simulink library "Feeder2_lib"  (Simulink 8.1)
settings: Solver=ode45  StartTime=0.0  StopTime=10.0  RelTol=1e-3
values from neighbouring files (symbols this model uses):
  DER_REL = xlsread('DER_relay.xlsx')    [relay_settings_init.m]
  Ts = 100E-6    (= 0.0001)    [BANSHEE_init.m]    (also in Ghost_init.m)
undefined symbols (not defined in the file or in its folder): CBID, Left, type, V
libraries: breaker_lib x22, powerlib x13, cables_lib x12, transformer_lib x10, Load_lib x8, ssn_lib x7, BESS_lib x2, relay_modbus_lib x2, rtio_generic_modbus x2, rtlab x2
settings Model: Creator=re25624  LastModifiedBy=MGC3

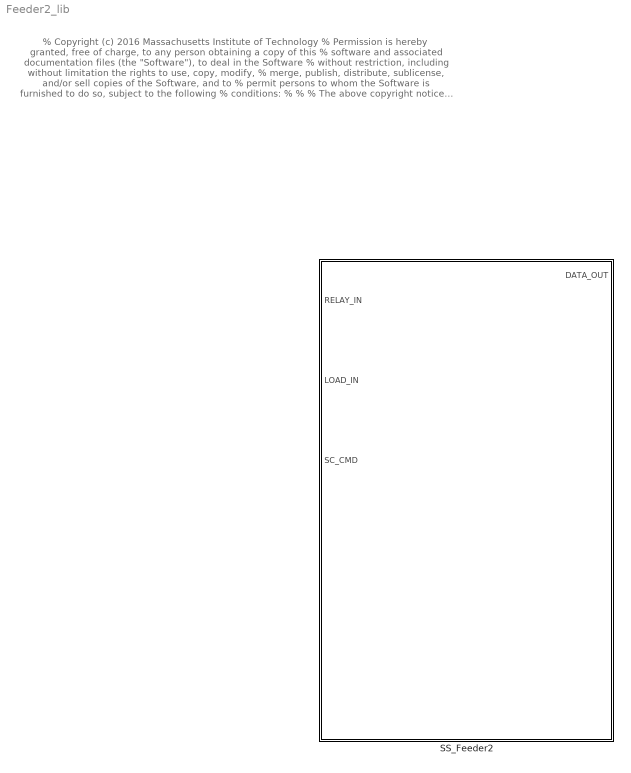
== system Feeder2_lib ==
  note: % Copyright (c) 2016 Massachusetts Institute of Technology
      | % Permission is hereby granted, free of charge, to any person obtaining a copy of this
      | % software and associated documentation files (the "Software"), to deal in the Software
      | % without restriction, including without limitation the rights to use, copy, modify,
      | % merge, publish, distribute, sublicense, and/or sell copies of the Software, and to
      | % permit persons to whom the Software is furnished to do so, subject to the following
      | % conditions:
      | %
      | %
      | % The above copyright notice and this permission notice shall be included in
      | % all copies or substantial portions of the Software.
      | %
      | % THE SOFTWARE IS PROVIDED "AS IS", WITHOUT WARRANTY OF ANY KIND, EXPRESS OR IMPLIED,
      | % INCLUDING BUT NOT LIMITED TO THE WARRANTIES OF MERCHANTABILITY, FITNESS FOR A
      | % PARTICULAR PURPOSE AND NONINFRINGEMENT. IN NO EVENT SHALL THE AUTHORS OR COPYRIGHT
      | % HOLDERS BE LIABLE FOR ANY CLAIM, DAMAGES OR OTHER LIABILITY, WHETHER IN AN ACTION
      | % OF CONTRACT, TORT OR OTHERWISE, ARISING FROM, OUT OF OR IN CONNECTION WITH THE
      | % SOFTWARE OR THE USE OR OTHER DEALINGS IN THE SOFTWARE.
      | %
      | %
      | %%
  SS_Feeder2 : Subsystem

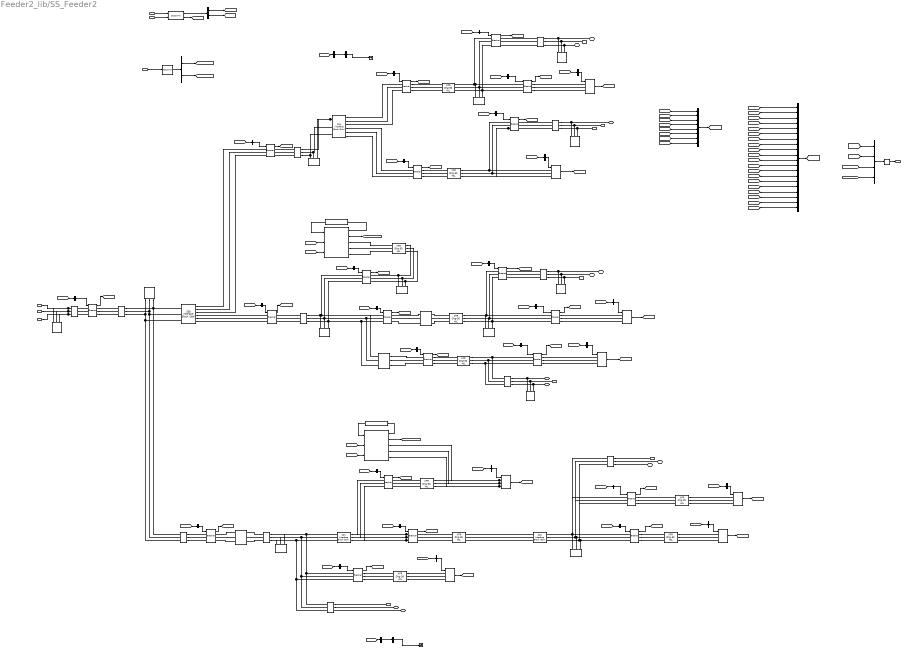
== system Feeder2_lib/SS_Feeder2 ==
  note: Fault6:
      | Fault Resistance: 0.1Ohm
      | Ground Resistance: 1.73Ohm
      | Snubber resistance: 1E6:
  note: Fault5:
      | Fault Resistance: 0.1Ohm
      | Ground Resistance: 1.73Ohm
      | Snubber resistance: 1E6:
  note: BESS SYSTEM
  note: % Copyright (c) 2016 Massachusetts Institute of Technology
      | % Permission is hereby granted, free of charge, to any person obtaining a copy of this
      | % software and associated documentation files (the "Software"), to deal in the Software
      | % without restriction, including without limitation the rights to use, copy, modify,
      | % merge, publish, distribute, sublicense, and/or sell copies of the Software, and to
      | % permit persons to whom the Software is furnished to do so, subject to the following
      | % conditions:
      | %
      | %
      | % The above copyright notice and this permission notice shall be included in
      | % all copies or substantial portions of the Software.
      | %
      | % THE SOFTWARE IS PROVIDED "AS IS", WITHOUT WARRANTY OF ANY KIND, EXPRESS OR IMPLIED,
      | % INCLUDING BUT NOT LIMITED TO THE WARRANTIES OF MERCHANTABILITY, FITNESS FOR A
      | % PARTICULAR PURPOSE AND NONINFRINGEMENT. IN NO EVENT SHALL THE AUTHORS OR COPYRIGHT
      | % HOLDERS BE LIABLE FOR ANY CLAIM, DAMAGES OR OTHER LIABILITY, WHETHER IN AN ACTION
      | % OF CONTRACT, TORT OR OTHERWISE, ARISING FROM, OUT OF OR IN CONNECTION WITH THE
      | % SOFTWARE OR THE USE OR OTHER DEALINGS IN THE SOFTWARE.
      | %
      | %
      | %%
  note: connect to F1
  note: PV SYSTEM
  note: connect to F3
  note: connect to F3
  note: connect to F3
  note: connect to F1
  note: connect to F1
  RELAY_IN : Inport
  LOAD_IN : Inport  Port=2
  SC_CMD : Inport  Port=3
  1000 kVA1 : transformer_lib/XFR DYg-30 HIL  Rating=1000  Vp=13800  Vs=480  Z=5.56  XR=4.49
  1000 kVA2 : transformer_lib/XFR DYg-30 HIL  Rating=1000  Vp=4160  Vs=480  Z=5.56  XR=5.49
  1500 kVA : transformer_lib/XFR DYg-30 HIL  Rating=1500  Vp=4160  Vs=480  Z=5.56  XR=5.51
  2000 kVA2 : transformer_lib/XFR DYg-30 HIL  Rating=2000  Vp=13800  Vs=480  Z=5.75  XR=5.7
  2000 kVA3 : transformer_lib/XFR DYg-30 HIL  Rating=2000  Vp=13800  Vs=480  Z=5.75  XR=5.7
  2500 kVA : transformer_lib/XFR DYg-30 HIL  Rating=2500  Vp=13800  Vs=480  Z=5.56  XR=5.52
  2500 kVA1 : transformer_lib/XFR DYg-30 HIL  Rating=2500  Vp=13800  Vs=480  Z=5.56  XR=5.52
  3750 kVA : transformer_lib/XFR DYg-30 HIL  Rating=3750  Vp=13800  Vs=4160  Z=4.75  XR=11.4
  4/0AWG-Mutual : cables_lib/4//0AWG-Mutual  length=10  par_sets=1  ratio=3
  448 kvar inductor at 13.8kV  to cancel kvar produced by the stublines1 : powerlib/Elements/Three-Phase Parallel RLC Load  LConnTagsString=A|B|C  Configuration=Y (grounded)  NominalVoltage=13800  NominalFrequency=60  ActivePower=10e3  InductivePower=448e3  CapacitivePower=0  Measurements=None  LoadType=constant Z
  500 kVA : transformer_lib/XFR DYg-30 HIL  Rating=500  Vp=13800  Vs=208  Z=5  XR=4.9
  5000 kVA : transformer_lib/XFR DYg-30 HIL  Rating=5000  Vp=13800  Vs=480  Z=3  XR=5.44
  500kcmil-Mutual4 : cables_lib/500kcmil-Mutual  length=10  par_sets=1  ratio=3
  500kcmil-Mutual5 : cables_lib/500kcmil-Mutual  length=1000  par_sets=1  ratio=3
  500kcmil-Mutual8 : cables_lib/500kcmil-Mutual  length=100  par_sets=1  ratio=3
  6 kvar inductor at 480V  to cancel kvar produced by the stublines1 : powerlib/Elements/Three-Phase Parallel RLC Load  LConnTagsString=A|B|C  Configuration=Y (grounded)  NominalVoltage=480  NominalFrequency=60  ActivePower=1e3  InductivePower=6e3  CapacitivePower=0  Measurements=None  LoadType=constant Z
  6 kvar inductor at 480V  to cancel kvar produced by the stublines2 : powerlib/Elements/Three-Phase Parallel RLC Load  LConnTagsString=A|B|C  Configuration=Y (grounded)  NominalVoltage=480  NominalFrequency=60  ActivePower=1e3  InductivePower=6e3  CapacitivePower=0  Measurements=None  LoadType=constant Z
  6 kvar inductor at 480V  to cancel kvar produced by the stublines3 : powerlib/Elements/Three-Phase Parallel RLC Load  LConnTagsString=A|B|C  Configuration=Y (grounded)  NominalVoltage=480  NominalFrequency=60  ActivePower=1  InductivePower=6e3  CapacitivePower=0  Measurements=None  LoadType=constant Z
  6 kvar inductor at 480V  to cancel kvar produced by the stublines4 : powerlib/Elements/Three-Phase Parallel RLC Load  LConnTagsString=A|B|C  Configuration=Y (grounded)  NominalVoltage=480  NominalFrequency=60  ActivePower=1  InductivePower=9e3  CapacitivePower=0  Measurements=None  LoadType=constant Z
  Bus Creator2 : BusCreator
  Bus Creator3 : BusCreator  Inputs=8
  Bus Creator5 : BusCreator  Inputs=20
  Bus Selector1 : BusSelector  OutputSignals=F2_CB_4
  Bus Selector10 : BusSelector  OutputSignals=I4
  Bus Selector11 : BusSelector  OutputSignals=F2_CB_11
  Bus Selector12 : BusSelector  OutputSignals=F2_CB_15
  Bus Selector13 : BusSelector  OutputSignals=F2_CB_3
  Bus Selector14 : BusSelector  OutputSignals=F2_CB_14
  Bus Selector15 : BusSelector  OutputSignals=F2_CB_17
  Bus Selector16 : BusSelector  OutputSignals=F2_CB_16
  Bus Selector17 : BusSelector  OutputSignals=F2_CB_13
  Bus Selector18 : BusSelector  OutputSignals=F2_CB_10
  Bus Selector19 : BusSelector  OutputSignals=F2_CB_9
  Bus Selector2 : BusSelector  OutputSignals=F2_CB_2
  Bus Selector20 : BusSelector  OutputSignals=F2_CB_12
  Bus Selector21 : BusSelector  OutputSignals=F2_CB_5
  Bus Selector22 : BusSelector  OutputSignals=F2_CB_7
  Bus Selector23 : BusSelector  OutputSignals=F2_CB_8
  Bus Selector24 : BusSelector  OutputSignals=F2_CB_6
  Bus Selector25 : BusSelector  OutputSignals=F2_CB_1
  Bus Selector26 : BusSelector  OutputSignals=F2_CB_18
  Bus Selector27 : BusSelector  OutputSignals=F2_CB_19
  Bus Selector28 : BusSelector  OutputSignals=ESS1_ctrl,PV1_ctrl
  Bus Selector29 : BusSelector  OutputSignals=fault
  Bus Selector3 : BusSelector  OutputSignals=P5
  Bus Selector30 : BusSelector  OutputSignals=LoadProfile,TestSeq
  Bus Selector31 : BusSelector  OutputSignals=loc6
  Bus Selector32 : BusSelector  OutputSignals=fault
  Bus Selector33 : BusSelector  OutputSignals=loc5
  Bus Selector36 : BusSelector  OutputSignals=F2_PCC
  Bus Selector4 : BusSelector  OutputSignals=C4
  Bus Selector5 : BusSelector  OutputSignals=I5
  Bus Selector6 : BusSelector  OutputSignals=P2
  Bus Selector7 : BusSelector  OutputSignals=C3
  Bus Selector8 : BusSelector  OutputSignals=P3
  Bus Selector9 : BusSelector  OutputSignals=I3
  C{1..2,204..206} (5 alike) : cables_lib/500kcmil-Mutual  length=10  par_sets=1  ratio=3
  C201 : cables_lib/4//0AWG-Mutual  length=5500  par_sets=1  ratio=3
  C202 : cables_lib/500kcmil-Mutual  length=2000  par_sets=1  ratio=3
  C203 : cables_lib/500kcmil-Mutual  length=3000  par_sets=1  ratio=3
  Critical_3 : Load_lib/Dynamic_Load  V=480  kVA=1000  PF=0.9  Ts=Ts
  Critical_4 : Load_lib/Dynamic_Load  V=480  kVA=1000  PF=0.9  Ts=Ts
  ESS1 : Subsystem
  ESS1_Modbus : rtio_generic_modbus/Modbus device  conf_name=ESS1_modbus.opal  conf_name_mask=ESS1_modbus.xls  sample_time=Ts
  F2_CB_{1..19} (19 alike) : breaker_lib/Breaker  Ts=Ts  mech_delay=cb_mech_delay
  F2_PCC : breaker_lib/Breaker  Ts=Ts  mech_delay=cb_mech_delay
  Interruptible_3 : Load_lib/Dynamic_Load  V=208  kVA=300  PF=0.9  Ts=Ts
  Interruptible_4 : Load_lib/Dynamic_Load  V=480  kVA=600  PF=0.9  Ts=Ts
  Interruptible_5 : Load_lib/Dynamic_Load  V=480  kVA=400  PF=0.9  Ts=Ts
  Losses{1,3..4,6,8} (5 alike) : powerlib/Elements/Three-Phase Parallel RLC Load  LConnTagsString=A|B|C  Configuration=Y (grounded)  NominalVoltage=13800  NominalFrequency=60  ActivePower=1e3  InductivePower=0  CapacitivePower=0  Measurements=None  LoadType=constant Z
  Losses2 : powerlib/Elements/Three-Phase Parallel RLC Load  LConnTagsString=A|B|C  Configuration=Y (grounded)  NominalVoltage=480  NominalFrequency=60  ActivePower=1e3  InductivePower=0  CapacitivePower=0  Measurements=None  LoadType=constant Z
  Losses5 : powerlib/Elements/Three-Phase Parallel RLC Load  LConnTagsString=A|B|C  Configuration=Y (grounded)  NominalVoltage=480  NominalFrequency=60  ActivePower=1e3  InductivePower=0  CapacitivePower=0  Measurements=None  LoadType=constant Z
  Losses7 : powerlib/Elements/Three-Phase Parallel RLC Load  LConnTagsString=A|B|C  Configuration=Y (grounded)  NominalVoltage=4160  NominalFrequency=60  ActivePower=1e3  InductivePower=0  CapacitivePower=0  Measurements=None  LoadType=constant Z
  Memory : Memory
  OpComm1 : rtlab/OpComm  nbport=2  groupe_acq=1  subsys_rate=0  st=0  Synchronization=on  Interpolation=on  Threshold=1.0  Missed_Data=off  Sim_Time=off  Samples=off  dynSigOut=off  from_console=0  warning_done=off  writeOpCommFile=off  Offset=off
  OpComm2 : rtlab/OpComm  nbport=1  groupe_acq=1  subsys_rate=0  st=0  Synchronization=on  Interpolation=on  Threshold=1.0  Missed_Data=off  Sim_Time=off  Samples=off  dynSigOut=off  from_console=1  warning_done=off  writeOpCommFile=off  Offset=off
  PV1_Modbus : rtio_generic_modbus/Modbus device  conf_name=PV1_modbus.opal  conf_name_mask=PV1_modbus.xls  sample_time=Ts
  PV2 : Subsystem
  Priority_2 : Load_lib/Dynamic_Load  V=480  kVA=1000  PF=0.9  Ts=Ts
  Priority_3 : Load_lib/Dynamic_Load  V=480  kVA=1000  PF=0.9  Ts=Ts
  Priority_5 : Load_lib/Dynamic_Load  V=480  kVA=700  PF=0.9  Ts=Ts
  SSN Interface Block (3ph){1,3,5,9..10} (5 alike) : ssn_lib/SSN Interface Block (3ph)  nb_phase=3  nb_port=2  p1_type=V-type(Left)  p2_type=V-type (Right)  p3_type=V-type(Left)  p4_type=V-type(Left)  p5_type=V-type(Left)  p6_type=V-type(Left)  p7_type=V-type(Left)  p8_type=V-type(Left)  p9_type=V-type(Left)  p10_type=V-type(Left)  p11_type=V-type(Left)  p12_type=V-type(Left)  p13_type=V-type(Left)  p14_type=V-type(Left)  p15_type=V-type(Left)  p16_type=V-type(Left)  I_port_shunt_resistance=1e9
  SSN Interface Block (3ph)2 : ssn_lib/SSN Interface Block (3ph)  nb_phase=3  nb_port=3  p1_type=V-type(Left)  p2_type=V-type (Right)  p3_type=V-type (Right)  p4_type=V-type(Left)  p5_type=V-type(Left)  p6_type=V-type(Left)  p7_type=V-type(Left)  p8_type=V-type(Left)  p9_type=V-type(Left)  p10_type=V-type(Left)  p11_type=V-type(Left)  p12_type=V-type(Left)  p13_type=V-type(Left)  p14_type=V-type(Left)  p15_type=V-type(Left)  p16_type=V-type(Left)  I_port_shunt_resistance=1e9
  SSN Interface Block (3ph)4 : ssn_lib/SSN Interface Block (3ph)  nb_phase=3  nb_port=3  p1_type=V-type(Left)  p2_type=V-type (Right)  p3_type=V-type (Right)  p4_type=V-type(Left)  p5_type=V-type(Left)  p6_type=V-type(Left)  p7_type=V-type(Left)  p8_type=V-type(Left)  p9_type=V-type(Left)  p10_type=V-type(Left)  p11_type=V-type(Left)  p12_type=V-type(Left)  p13_type=V-type(Left)  p14_type=V-type(Left)  p15_type=V-type(Left)  p16_type=V-type(Left)  I_port_shunt_resistance=1e9
  Terminator : Terminator
  Terminator1 : Terminator
  A_CB_13 : PMIOPort  Port=1  Side=Right
  B_CB_13 : PMIOPort  Port=2  Side=Right
  C_CB_13 : PMIOPort  Port=3  Side=Right
  A_CB_17 : PMIOPort  Port=4  Side=Right
  B_CB_17 : PMIOPort  Port=5  Side=Right
  C_CB_17 : PMIOPort  Port=6  Side=Right
  A_CB_16 : PMIOPort  Port=7  Side=Right
  B_CB_16 : PMIOPort  Port=8  Side=Right
  C_CB_16 : PMIOPort  Port=9  Side=Right
  A_CB_9 : PMIOPort  Port=10  Side=Right
  B_CB_9 : PMIOPort  Port=11  Side=Right
  C_CB_9 : PMIOPort  Port=12  Side=Right
  A_CB_7 : PMIOPort  Port=13  Side=Right
  B_CB_7 : PMIOPort  Port=14  Side=Right
  C_CB_7 : PMIOPort  Port=15  Side=Right
  A_CB_1 : PMIOPort  Port=16  Side=Right
  B_CB_1 : PMIOPort  Port=17  Side=Right
  C_CB_1 : PMIOPort  Port=18  Side=Right
  PCC_A : PMIOPort  Port=19  Side=Left
  PCC_B : PMIOPort  Port=20  Side=Left
  PCC_C : PMIOPort  Port=21  Side=Left
  DATA_OUT : Outport
  wires:
  Bus Selector33/1 -> Terminator/1  "<loc5>"
  Bus Selector32/1 -> Bus Selector33/1  "<fault>"
  [TestSeq] -> Bus Selector32/1
  Bus Selector31/1 -> Terminator1/1  "<loc6>"
  Bus Selector29/1 -> Bus Selector31/1  "<fault>"
  [TestSeq] -> Bus Selector29/1
  [TestSeq] -> ESS1/3(testseq)
  [TestSeq] -> PV2/2(testseq)
  Bus Selector30/2 -> [TestSeq]  "<TestSeq>"
  Bus Selector30/1 -> [LOAD_IN]  "<LoadProfile>"
  OpComm1/1 -> Bus Selector30/1
  ESS1_Modbus/1 -> ESS1/1(modbus_in)
  ESS1/1(modbus_out) -> ESS1_Modbus/1
  ESS1/2(meas) -> [ESS_DATA]
  [ESS] -> ESS1/2(console)
  PV2/2(meas) -> [PV_DATA]
  PV2/1(modbus_out) -> PV1_Modbus/1
  [PV] -> PV2/3(console)
  PV1_Modbus/1 -> PV2/1(modbus_in)
  Bus Selector28/2 -> [PV]  "<PV1_ctrl>"
  Bus Selector28/1 -> [ESS]  "<ESS1_ctrl>"
  [PV_DATA] -> Bus Creator2/4  "PV_DATA"
  [ESS_DATA] -> Bus Creator2/3  "ESS_DATA"
  Bus Selector36/1 -> F2_PCC/1  "<F2_PCC>"
  [RELAY_IN] -> Bus Selector36/1
  F2_CB_18/1 -> [F2_CB_18]
  [LOAD_DATA] -> Bus Creator2/2  "LOAD_DATA"
  [CB_DATA] -> Bus Creator2/1  "CB_DATA"
  Bus Creator5/1 -> [CB_DATA]
  Bus Creator2/1 -> Memory/1
  OpComm2/1 -> Bus Selector28/1
  Memory/1 -> DATA_OUT/1
  SC_CMD/1 -> OpComm2/1
  Bus Selector27/1 -> F2_CB_19/1  "<F2_CB_19>"
  [RELAY_IN] -> Bus Selector27/1
  F2_CB_19/1 -> [F2_CB_19]
  [F2_CB_19] -> Bus Creator5/19  "F2_CB_19"
  [F2_CB_18] -> Bus Creator5/18  "F2_CB_18"
  Bus Selector26/1 -> F2_CB_18/1  "<F2_CB_18>"
  [RELAY_IN] -> Bus Selector26/1
  Bus Selector1/1 -> F2_CB_4/1  "<F2_CB_4>"
  [RELAY_IN] -> Bus Selector1/1
  F2_CB_4/1 -> [F2_CB_4]
  [F2_PCC] -> Bus Creator5/20  "F2_PCC"
  F2_PCC/1 -> [F2_PCC]
  F2_CB_16/1 -> [F2_CB_16]
  F2_CB_12/1 -> [F2_CB_12]
  Bus Selector15/1 -> F2_CB_17/1  "<F2_CB_17>"
  [F2_CB_17] -> Bus Creator5/17  "F2_CB_17"
  Bus Selector23/1 -> F2_CB_8/1  "<F2_CB_8>"
  Bus Selector24/1 -> F2_CB_6/1  "<F2_CB_6>"
  Bus Selector22/1 -> F2_CB_7/1  "<F2_CB_7>"
  Bus Selector21/1 -> F2_CB_5/1  "<F2_CB_5>"
  Bus Selector25/1 -> F2_CB_1/1  "<F2_CB_1>"
  Bus Selector12/1 -> F2_CB_15/1  "<F2_CB_15>"
  Bus Selector16/1 -> F2_CB_16/1  "<F2_CB_16>"
  Bus Selector14/1 -> F2_CB_14/1  "<F2_CB_14>"
  Bus Selector20/1 -> F2_CB_12/1  "<F2_CB_12>"
  Bus Selector17/1 -> F2_CB_13/1  "<F2_CB_13>"
  Bus Selector19/1 -> F2_CB_9/1  "<F2_CB_9>"
  Bus Selector18/1 -> F2_CB_10/1  "<F2_CB_10>"
  Bus Selector11/1 -> F2_CB_11/1  "<F2_CB_11>"
  Bus Selector2/1 -> F2_CB_2/1  "<F2_CB_2>"
  [RELAY_IN] -> Bus Selector25/1
  [RELAY_IN] -> Bus Selector24/1
  [RELAY_IN] -> Bus Selector23/1
  [RELAY_IN] -> Bus Selector22/1
  [RELAY_IN] -> Bus Selector21/1
  [RELAY_IN] -> Bus Selector20/1
  [RELAY_IN] -> Bus Selector19/1
  [RELAY_IN] -> Bus Selector18/1
  [RELAY_IN] -> Bus Selector17/1
  [RELAY_IN] -> Bus Selector16/1
  [RELAY_IN] -> Bus Selector15/1
  [RELAY_IN] -> Bus Selector14/1
  [RELAY_IN] -> Bus Selector12/1
  [RELAY_IN] -> Bus Selector11/1
  [RELAY_IN] -> Bus Selector2/1
  [RELAY_IN] -> Bus Selector13/1
  Bus Selector13/1 -> F2_CB_3/1  "<F2_CB_3>"
  OpComm1/2 -> [RELAY_IN]
  RELAY_IN/1 -> OpComm1/2
  [F2_CB_16] -> Bus Creator5/16  "F2_CB_16"
  [F2_CB_15] -> Bus Creator5/15  "F2_CB_15"
  [F2_CB_13] -> Bus Creator5/13  "F2_CB_13"
  [F2_CB_10] -> Bus Creator5/10  "F2_CB_10"
  [F2_CB_12] -> Bus Creator5/12  "F2_CB_12"
  [F2_CB_8] -> Bus Creator5/8  "F2_CB_8"
  [F2_CB_5] -> Bus Creator5/5  "F2_CB_5"
  [F2_CB_14] -> Bus Creator5/14  "F2_CB_14"
  [F2_CB_11] -> Bus Creator5/11  "F2_CB_11"
  [F2_CB_7] -> Bus Creator5/7  "F2_CB_7"
  [F2_CB_9] -> Bus Creator5/9  "F2_CB_9"
  [F2_CB_4] -> Bus Creator5/4  "F2_CB_4"
  [F2_CB_6] -> Bus Creator5/6  "F2_CB_6"
  [F2_CB_3] -> Bus Creator5/3  "F2_CB_3"
  [F2_CB_2] -> Bus Creator5/2  "F2_CB_2"
  [F2_CB_1] -> Bus Creator5/1  "F2_CB_1"
  F2_CB_13/1 -> [F2_CB_13]
  F2_CB_10/1 -> [F2_CB_10]
  F2_CB_14/1 -> [F2_CB_14]
  F2_CB_17/1 -> [F2_CB_17]
  F2_CB_15/1 -> [F2_CB_15]
  F2_CB_11/1 -> [F2_CB_11]
  F2_CB_3/1 -> [F2_CB_3]
  F2_CB_9/1 -> [F2_CB_9]
  F2_CB_8/1 -> [F2_CB_8]
  F2_CB_5/1 -> [F2_CB_5]
  F2_CB_7/1 -> [F2_CB_7]
  F2_CB_6/1 -> [F2_CB_6]
  F2_CB_1/1 -> [F2_CB_1]
  F2_CB_2/1 -> [F2_CB_2]
  [LOAD_P5] -> Bus Creator3/8  "F2_P5"
  [LOAD_P3] -> Bus Creator3/7  "F2_P3"
  [LOAD_I3] -> Bus Creator3/3  "F2_I3"
  [LOAD_C4] -> Bus Creator3/2  "F2_C4"
  [LOAD_I5] -> Bus Creator3/5  "F2_I5"
  [LOAD_P2] -> Bus Creator3/6  "F2_P2"
  [LOAD_I4] -> Bus Creator3/4  "F2_I4"
  Bus Creator3/1 -> [LOAD_DATA]  "LOAD"
  [LOAD_C3] -> Bus Creator3/1  "F2_C3"
  Interruptible_4/1 -> [LOAD_I4]
  Priority_3/1 -> [LOAD_P3]
  Interruptible_3/1 -> [LOAD_I3]
  Critical_3/1 -> [LOAD_C3]
  Priority_2/1 -> [LOAD_P2]
  Interruptible_5/1 -> [LOAD_I5]
  Priority_5/1 -> [LOAD_P5]
  Critical_4/1 -> [LOAD_C4]
  Bus Selector9/1 -> Interruptible_3/1  "<I3>"
  Bus Selector10/1 -> Interruptible_4/1  "<I4>"
  Bus Selector8/1 -> Priority_3/1  "<P3>"
  Bus Selector7/1 -> Critical_3/1  "<C3>"
  Bus Selector6/1 -> Priority_2/1  "<P2>"
  Bus Selector5/1 -> Interruptible_5/1  "<I5>"
  Bus Selector4/1 -> Critical_4/1  "<C4>"
  Bus Selector3/1 -> Priority_5/1  "<P5>"
  [LOAD_IN] -> Bus Selector10/1
  [LOAD_IN] -> Bus Selector9/1
  [LOAD_IN] -> Bus Selector8/1
  [LOAD_IN] -> Bus Selector7/1
  [LOAD_IN] -> Bus Selector6/1
  [LOAD_IN] -> Bus Selector5/1
  [LOAD_IN] -> Bus Selector4/1
  [LOAD_IN] -> Bus Selector3/1
  LOAD_IN/1 -> OpComm1/1
  connections:
  C_CB_1/RConn1 -- C2/RConn3
  F2_CB_8/LConn1 -- Losses7/LConn1 -- SSN Interface Block (3ph)1/RConn1 -- C1/LConn1 -- F2_CB_4/LConn1
  C1/RConn2 -- B_CB_7/RConn1
  C1/RConn1 -- A_CB_7/RConn1
  C1/RConn3 -- C_CB_7/RConn1
  C2/RConn2 -- B_CB_1/RConn1
  C2/RConn1 -- A_CB_1/RConn1
  F2_CB_8/LConn2 -- Losses7/LConn2 -- SSN Interface Block (3ph)1/RConn2 -- F2_CB_4/LConn2 -- C1/LConn2
  F2_CB_8/LConn3 -- Losses7/LConn3 -- SSN Interface Block (3ph)1/RConn3 -- F2_CB_4/LConn3 -- C1/LConn3
  F2_CB_6/LConn2 -- Losses8/LConn2 -- C201/RConn2 -- SSN Interface Block (3ph)5/LConn2 -- C2/LConn2
  C2/LConn1 -- F2_CB_6/LConn1 -- Losses8/LConn3 -- C201/RConn1 -- SSN Interface Block (3ph)5/LConn1
  C2/LConn3 -- F2_CB_6/LConn3 -- Losses8/LConn1 -- C201/RConn3 -- SSN Interface Block (3ph)5/LConn3
  PV2/RConn2 -- 5000 kVA/RConn2
  PV2/RConn3 -- 5000 kVA/RConn3
  PV2/RConn1 -- 5000 kVA/RConn1
  SSN Interface Block (3ph)1/LConn1 -- 3750 kVA/RConn1
  SSN Interface Block (3ph)1/LConn2 -- 3750 kVA/RConn2
  SSN Interface Block (3ph)1/LConn3 -- 3750 kVA/RConn3
  F2_CB_7/LConn3 -- F2_CB_5/LConn3 -- SSN Interface Block (3ph)5/RConn3
  F2_CB_7/LConn1 -- F2_CB_5/LConn1 -- SSN Interface Block (3ph)5/RConn1
  F2_CB_7/LConn2 -- F2_CB_5/LConn2 -- SSN Interface Block (3ph)5/RConn2
  C201/LConn3 -- SSN Interface Block (3ph)10/RConn3
  C201/LConn1 -- SSN Interface Block (3ph)10/RConn1
  C201/LConn2 -- SSN Interface Block (3ph)10/RConn2
  SSN Interface Block (3ph)10/LConn1 -- F2_CB_1/RConn1
  SSN Interface Block (3ph)10/LConn2 -- F2_CB_1/RConn2
  SSN Interface Block (3ph)10/LConn3 -- F2_CB_1/RConn3
  4/0AWG-Mutual/RConn3 -- F2_CB_1/LConn3
  4/0AWG-Mutual/RConn1 -- F2_CB_1/LConn1
  4/0AWG-Mutual/RConn2 -- F2_CB_1/LConn2
  500kcmil-Mutual5/LConn3 -- 448 kvar inductor at 13.8kV  to cancel kvar produced by the stublines1/LConn3 -- PCC_C/RConn1
  500kcmil-Mutual5/LConn1 -- 448 kvar inductor at 13.8kV  to cancel kvar produced by the stublines1/LConn1 -- PCC_A/RConn1
  500kcmil-Mutual5/LConn2 -- 448 kvar inductor at 13.8kV  to cancel kvar produced by the stublines1/LConn2 -- PCC_B/RConn1
  F2_CB_18/RConn1 -- Priority_5/LConn1
  F2_PCC/LConn1 -- 500kcmil-Mutual5/RConn1
  F2_PCC/LConn2 -- 500kcmil-Mutual5/RConn2
  F2_PCC/LConn3 -- 500kcmil-Mutual5/RConn3
  F2_PCC/RConn3 -- 500kcmil-Mutual8/LConn3
  F2_PCC/RConn2 -- 500kcmil-Mutual8/LConn2
  F2_PCC/RConn1 -- 500kcmil-Mutual8/LConn1
  6 kvar inductor at 480V  to cancel kvar produced by the stublines4/LConn2 -- 500kcmil-Mutual4/RConn2 -- B_CB_9/RConn1
  6 kvar inductor at 480V  to cancel kvar produced by the stublines4/LConn3 -- 500kcmil-Mutual4/RConn3 -- C_CB_9/RConn1
  6 kvar inductor at 480V  to cancel kvar produced by the stublines4/LConn1 -- 500kcmil-Mutual4/RConn1 -- A_CB_9/RConn1
  500 kVA/RConn1 -- Interruptible_3/LConn1
  500 kVA/RConn3 -- Interruptible_3/LConn3
  500 kVA/RConn2 -- Interruptible_3/LConn2
  1000 kVA2/RConn3 -- Interruptible_4/LConn3
  1000 kVA2/RConn2 -- Interruptible_4/LConn2
  1000 kVA2/RConn1 -- Interruptible_4/LConn1
  Critical_3/LConn2 -- ESS1/RConn2 -- 2500 kVA/RConn2
  Critical_3/LConn3 -- ESS1/RConn3 -- 2500 kVA/RConn3
  Critical_3/LConn1 -- ESS1/RConn1 -- 2500 kVA/RConn1
  SSN Interface Block (3ph)2/RConn4 -- F2_CB_14/LConn1
  SSN Interface Block (3ph)2/RConn5 -- F2_CB_14/LConn2
  SSN Interface Block (3ph)2/RConn6 -- F2_CB_14/LConn3
  SSN Interface Block (3ph)2/RConn3 -- F2_CB_15/LConn3
  SSN Interface Block (3ph)2/RConn2 -- F2_CB_15/LConn2
  SSN Interface Block (3ph)2/RConn1 -- F2_CB_15/LConn1
  C202/LConn3 -- F2_CB_2/RConn3
  C202/LConn1 -- F2_CB_2/RConn1
  C202/LConn2 -- F2_CB_2/RConn2
  SSN Interface Block (3ph)4/RConn4 -- F2_CB_2/LConn1
  SSN Interface Block (3ph)4/RConn6 -- F2_CB_2/LConn3
  SSN Interface Block (3ph)4/RConn5 -- F2_CB_2/LConn2
  F2_CB_4/RConn1 -- 1500 kVA/LConn1
  F2_CB_4/RConn2 -- 1500 kVA/LConn2
  F2_CB_4/RConn3 -- 1500 kVA/LConn3
  1500 kVA/RConn1 -- Priority_3/LConn1
  1500 kVA/RConn2 -- Priority_3/LConn2
  1500 kVA/RConn3 -- Priority_3/LConn3
  6 kvar inductor at 480V  to cancel kvar produced by the stublines3/LConn1 -- C206/RConn1 -- A_CB_13/RConn1
  6 kvar inductor at 480V  to cancel kvar produced by the stublines3/LConn2 -- C206/RConn2 -- B_CB_13/RConn1
  6 kvar inductor at 480V  to cancel kvar produced by the stublines3/LConn3 -- C206/RConn3 -- C_CB_13/RConn1
  C206/LConn1 -- F2_CB_13/RConn1
  C206/LConn2 -- F2_CB_13/RConn2
  C206/LConn3 -- F2_CB_13/RConn3
  6 kvar inductor at 480V  to cancel kvar produced by the stublines2/LConn1 -- C205/RConn1 -- A_CB_17/RConn1
  6 kvar inductor at 480V  to cancel kvar produced by the stublines2/LConn2 -- C205/RConn2 -- B_CB_17/RConn1
  6 kvar inductor at 480V  to cancel kvar produced by the stublines2/LConn3 -- C205/RConn3 -- C_CB_17/RConn1
  C205/LConn2 -- F2_CB_17/RConn2
  C205/LConn1 -- F2_CB_17/RConn1
  C205/LConn3 -- F2_CB_17/RConn3
  6 kvar inductor at 480V  to cancel kvar produced by the stublines1/LConn1 -- C204/RConn1 -- A_CB_16/RConn1
  6 kvar inductor at 480V  to cancel kvar produced by the stublines1/LConn2 -- C204/RConn2 -- B_CB_16/RConn1
  6 kvar inductor at 480V  to cancel kvar produced by the stublines1/LConn3 -- C204/RConn3 -- C_CB_16/RConn1
  C204/LConn2 -- F2_CB_16/RConn2
  C204/LConn1 -- F2_CB_16/RConn1
  C204/LConn3 -- F2_CB_16/RConn3
  SSN Interface Block (3ph)3/RConn1 -- F2_CB_9/LConn1
  SSN Interface Block (3ph)3/RConn3 -- F2_CB_9/LConn3
  SSN Interface Block (3ph)3/RConn2 -- F2_CB_9/LConn2
  F2_CB_19/RConn3 -- Priority_2/LConn3
  F2_CB_19/RConn2 -- Priority_2/LConn2
  F2_CB_19/RConn1 -- Priority_2/LConn1
  F2_CB_18/RConn3 -- Priority_5/LConn3
  F2_CB_18/RConn2 -- Priority_5/LConn2
  F2_CB_19/LConn3 -- 500kcmil-Mutual4/LConn3 -- 2500 kVA1/RConn3
  F2_CB_19/LConn1 -- 500kcmil-Mutual4/LConn1 -- 2500 kVA1/RConn1
  F2_CB_9/RConn2 -- 2500 kVA1/LConn2
  Losses6/LConn1 -- SSN Interface Block (3ph)4/LConn3 -- 4/0AWG-Mutual/LConn3 -- 500kcmil-Mutual8/RConn3
  Losses6/LConn2 -- 500kcmil-Mutual8/RConn2 -- 4/0AWG-Mutual/LConn2 -- SSN Interface Block (3ph)4/LConn2
  F2_CB_6/RConn1 -- 500 kVA/LConn1
  F2_CB_15/RConn2 -- 2000 kVA3/LConn2
  Losses3/LConn1 -- C202/RConn1 -- F2_CB_10/LConn1 -- SSN Interface Block (3ph)3/LConn1 -- F2_CB_11/LConn1
  3750 kVA/LConn1 -- F2_CB_7/RConn1
  3750 kVA/LConn2 -- F2_CB_7/RConn2
  2000 kVA2/RConn2 -- F2_CB_17/LConn2 -- Critical_4/LConn2
  Losses4/LConn3 -- 5000 kVA/LConn3 -- F2_CB_11/RConn3
  C203/LConn2 -- F2_CB_3/RConn2
  F2_CB_19/LConn2 -- 500kcmil-Mutual4/LConn2 -- 2500 kVA1/RConn2
  F2_CB_9/RConn1 -- 2500 kVA1/LConn1
  F2_CB_15/RConn3 -- 2000 kVA3/LConn3
  Losses4/LConn1 -- 5000 kVA/LConn1 -- F2_CB_11/RConn1
  F2_CB_17/LConn3 -- 2000 kVA2/RConn3 -- Critical_4/LConn3
  F2_CB_15/RConn1 -- 2000 kVA3/LConn1
  F2_CB_14/RConn1 -- 2000 kVA2/LConn1
  SSN Interface Block (3ph)9/LConn1 -- F2_CB_10/RConn1
  F2_CB_18/LConn1 -- Losses2/LConn1 -- 2000 kVA3/RConn1 -- F2_CB_16/LConn1
  2500 kVA/LConn2 -- F2_CB_5/RConn2
  2500 kVA/LConn3 -- F2_CB_5/RConn3
  2500 kVA/LConn1 -- F2_CB_5/RConn1
  SSN Interface Block (3ph)9/LConn2 -- F2_CB_10/RConn2
  C203/LConn1 -- F2_CB_3/RConn1
  C203/LConn3 -- F2_CB_3/RConn3
  3750 kVA/LConn3 -- F2_CB_7/RConn3
  Losses6/LConn3 -- SSN Interface Block (3ph)4/LConn1 -- 500kcmil-Mutual8/RConn1 -- 4/0AWG-Mutual/LConn1
  SSN Interface Block (3ph)3/LConn2 -- F2_CB_10/LConn2 -- Losses3/LConn2 -- F2_CB_11/LConn2 -- C202/RConn2
  2000 kVA2/RConn1 -- F2_CB_17/LConn1 -- Critical_4/LConn1
  Losses4/LConn2 -- 5000 kVA/LConn2 -- F2_CB_11/RConn2
  F2_CB_18/LConn3 -- 2000 kVA3/RConn3 -- Losses2/LConn3 -- F2_CB_16/LConn3
  F2_CB_6/RConn3 -- 500 kVA/LConn3
  F2_CB_10/LConn3 -- SSN Interface Block (3ph)3/LConn3 -- Losses3/LConn3 -- F2_CB_11/LConn3 -- C202/RConn3
  F2_CB_9/RConn3 -- 2500 kVA1/LConn3
  SSN Interface Block (3ph)9/LConn3 -- F2_CB_10/RConn3
  F2_CB_6/RConn2 -- 500 kVA/LConn2
  F2_CB_14/RConn2 -- 2000 kVA2/LConn2
  F2_CB_18/LConn2 -- 2000 kVA3/RConn2 -- Losses2/LConn2 -- F2_CB_16/LConn2
  F2_CB_14/RConn3 -- 2000 kVA2/LConn3
  SSN Interface Block (3ph)4/RConn2 -- F2_CB_3/LConn2
  SSN Interface Block (3ph)4/RConn1 -- F2_CB_3/LConn1
  SSN Interface Block (3ph)4/RConn3 -- F2_CB_3/LConn3
  F2_CB_8/RConn2 -- 1000 kVA2/LConn2
  F2_CB_8/RConn1 -- 1000 kVA2/LConn1
  F2_CB_8/RConn3 -- 1000 kVA2/LConn3
  1000 kVA1/LConn2 -- SSN Interface Block (3ph)9/RConn2
  1000 kVA1/LConn3 -- SSN Interface Block (3ph)9/RConn3
  1000 kVA1/LConn1 -- SSN Interface Block (3ph)9/RConn1
  F2_CB_12/RConn1 -- Interruptible_5/LConn1
  F2_CB_12/RConn2 -- Interruptible_5/LConn2
  F2_CB_12/RConn3 -- Interruptible_5/LConn3
  F2_CB_12/LConn3 -- 1000 kVA1/RConn3 -- F2_CB_13/LConn3 -- Losses5/LConn3
  F2_CB_12/LConn2 -- Losses5/LConn2 -- 1000 kVA1/RConn2 -- F2_CB_13/LConn2
  F2_CB_12/LConn1 -- Losses5/LConn1 -- 1000 kVA1/RConn1 -- F2_CB_13/LConn1
  Losses1/LConn1 -- C203/RConn3 -- SSN Interface Block (3ph)2/LConn3
  Losses1/LConn2 -- C203/RConn2 -- SSN Interface Block (3ph)2/LConn2
  SSN Interface Block (3ph)2/LConn1 -- Losses1/LConn3 -- C203/RConn1

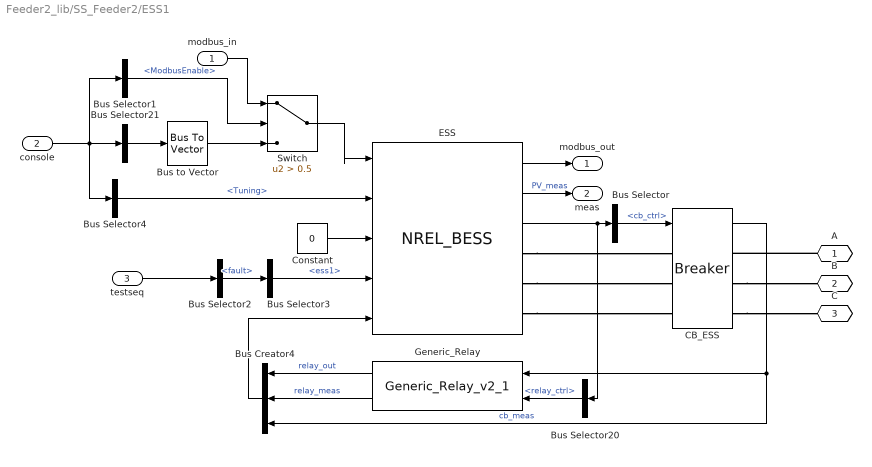
== system Feeder2_lib/SS_Feeder2/ESS1 ==
  modbus_in : Inport
  console : Inport  Port=2
  testseq : Inport  Port=3
  Bus Creator4 : BusCreator  Inputs=3
  Bus Selector : BusSelector  OutputSignals=cb_ctrl
  Bus Selector1 : BusSelector  OutputSignals=ModbusEnable
  Bus Selector2 : BusSelector  OutputSignals=fault
  Bus Selector20 : BusSelector  OutputSignals=relay_ctrl
  Bus Selector21 : BusSelector  OutputSignals=ModbusFromSC.Ctrl,ModbusFromSC.PCmd,ModbusFromSC.QCmd,ModbusFromSC.VoltCmd,ModbusFromSC.FreqCmd,ModbusFromSC.signal6,ModbusFromSC.signal7,ModbusFromSC.signal8  OutputAsBus=on
  Bus Selector3 : BusSelector  OutputSignals=ess1
  Bus Selector4 : BusSelector  OutputSignals=Tuning
  Bus to Vector : BusToVector
  CB_ESS : breaker_lib/Breaker  Ts=Ts  mech_delay=cb_mech_delay
  Constant : Constant  Value=0
  ESS : BESS_lib/NREL_BESS  InvType=ESS Inverter  Sn=3000  Vn=480  b_Vdc_nom=1000  b_kWh=600  b_esr=0.005  r_I_max=3  Tc=Ts  MbusPrecInc=off  ExtTuningEna=on
  Generic_Relay : relay_modbus_lib/Generic_Relay_v2_1  Ts=Ts  relay_settings=[DER_REL(CBID.ESS1,:)]
  Switch : Switch  Criteria=u2 > Threshold  Threshold=0.5
  A : PMIOPort  Port=1  Side=Right
  B : PMIOPort  Port=2  Side=Right
  C : PMIOPort  Port=3  Side=Right
  modbus_out : Outport
  meas : Outport  Port=2
  wires:
  Bus Selector4/1 -> ESS/2  "<Tuning>"
  Bus Selector/1 -> CB_ESS/1  "<cb_ctrl>"
  Bus Selector3/1 -> ESS/4  "<ess1>"
  Bus Selector2/1 -> Bus Selector3/1  "<fault>"
  testseq/1 -> Bus Selector2/1
  Constant/1 -> ESS/3
  Bus to Vector/1 -> Switch/3
  ESS/3 -> Bus Selector/1, Bus Selector20/1
  CB_ESS/1 -> Bus Creator4/3, Generic_Relay/1  "cb_meas"
  Switch/1 -> ESS/1
  Bus Selector21/1 -> Bus to Vector/1
  modbus_in/1 -> Switch/1
  ESS/1 -> modbus_out/1
  Bus Selector1/1 -> Switch/2  "<ModbusEnable>"
  console/1 -> Bus Selector21/1, Bus Selector1/1, Bus Selector4/1
  Bus Selector20/1 -> Generic_Relay/2  "<relay_ctrl>"
  Generic_Relay/1 -> Bus Creator4/1  "relay_out"
  ESS/2 -> meas/1  "PV_meas"
  Generic_Relay/2 -> Bus Creator4/2  "relay_meas"
  Bus Creator4/1 -> ESS/5
  connections:
  CB_ESS/RConn3 -- C/RConn1
  A/RConn1 -- CB_ESS/RConn1
  ESS/RConn1 -- CB_ESS/LConn1
  ESS/RConn3 -- CB_ESS/LConn3
  ESS/RConn2 -- CB_ESS/LConn2
  CB_ESS/RConn2 -- B/RConn1

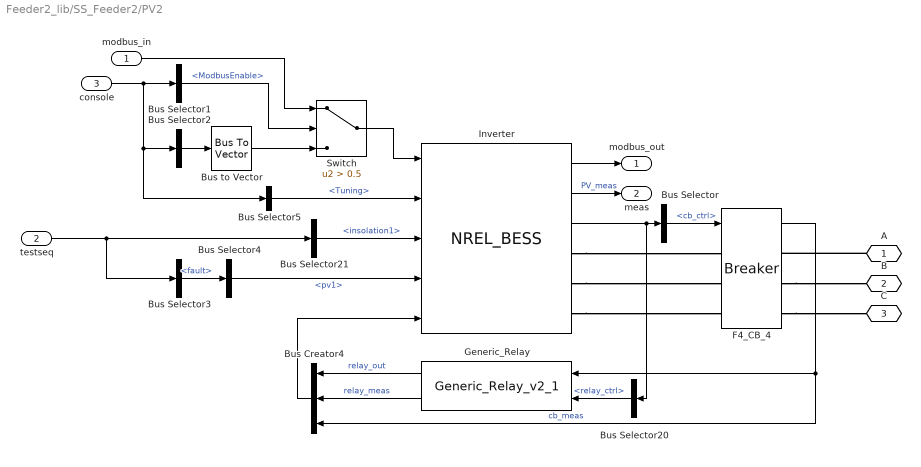
== system Feeder2_lib/SS_Feeder2/PV2 ==
  modbus_in : Inport
  testseq : Inport  Port=2
  console : Inport  Port=3
  Bus Creator4 : BusCreator  Inputs=3
  Bus Selector : BusSelector  OutputSignals=cb_ctrl
  Bus Selector1 : BusSelector  OutputSignals=ModbusEnable
  Bus Selector2 : BusSelector  OutputSignals=ModbusFromSC.Ctrl,ModbusFromSC.PCmd,ModbusFromSC.QCmd,ModbusFromSC.VoltCmd,ModbusFromSC.FreqCmd,ModbusFromSC.signal6,ModbusFromSC.signal7,ModbusFromSC.signal8  OutputAsBus=on
  Bus Selector20 : BusSelector  OutputSignals=relay_ctrl
  Bus Selector21 : BusSelector  OutputSignals=pv.insolation1
  Bus Selector3 : BusSelector  OutputSignals=fault
  Bus Selector4 : BusSelector  OutputSignals=pv1
  Bus Selector5 : BusSelector  OutputSignals=Tuning
  Bus to Vector : BusToVector
  F4_CB_4 : breaker_lib/Breaker  Ts=Ts  mech_delay=cb_mech_delay
  Generic_Relay : relay_modbus_lib/Generic_Relay_v2_1  Ts=Ts  relay_settings=[DER_REL(CBID.PV1,:)]
  Inverter : BESS_lib/NREL_BESS  InvType=PV Inverter  Sn=5000  Vn=480  b_Vdc_nom=1000  b_kWh=1000  b_esr=0.002  r_I_max=1.2  Tc=Ts  MbusPrecInc=off  ExtTuningEna=on
  Switch : Switch  Criteria=u2 > Threshold  Threshold=0.5
  A : PMIOPort  Port=1  Side=Right
  B : PMIOPort  Port=2  Side=Right
  C : PMIOPort  Port=3  Side=Right
  modbus_out : Outport
  meas : Outport  Port=2
  wires:
  Bus Selector5/1 -> Inverter/2  "<Tuning>"
  Bus Selector/1 -> F4_CB_4/1  "<cb_ctrl>"
  Bus Selector4/1 -> Inverter/4  "<pv1>"
  Bus Selector3/1 -> Bus Selector4/1  "<fault>"
  testseq/1 -> Bus Selector21/1, Bus Selector3/1
  Bus Selector2/1 -> Bus to Vector/1
  Bus Selector1/1 -> Switch/2  "<ModbusEnable>"
  console/1 -> Bus Selector1/1, Bus Selector2/1, Bus Selector5/1
  Bus to Vector/1 -> Switch/3
  Bus Selector21/1 -> Inverter/3  "<insolation1>"
  Bus Creator4/1 -> Inverter/5
  Generic_Relay/2 -> Bus Creator4/2  "relay_meas"
  Inverter/2 -> meas/1  "PV_meas"
  Generic_Relay/1 -> Bus Creator4/1  "relay_out"
  Bus Selector20/1 -> Generic_Relay/2  "<relay_ctrl>"
  Inverter/1 -> modbus_out/1
  modbus_in/1 -> Switch/1
  Switch/1 -> Inverter/1
  F4_CB_4/1 -> Generic_Relay/1, Bus Creator4/3  "cb_meas"
  Inverter/3 -> Bus Selector/1, Bus Selector20/1
  connections:
  F4_CB_4/RConn2 -- B/RConn1
  Inverter/RConn2 -- F4_CB_4/LConn2
  Inverter/RConn3 -- F4_CB_4/LConn3
  Inverter/RConn1 -- F4_CB_4/LConn1
  A/RConn1 -- F4_CB_4/RConn1
  F4_CB_4/RConn3 -- C/RConn1
